simulink model "Test_Model_HR12_2016"  (R2016b)
settings: Solver=FixedStepAuto  StartTime=0.0  StopTime=length(ipoint)  FixedStep=dt  RelTol=1e-3
values from neighbouring files (symbols this model uses):
  Cbx_cyl_fill_efy_intk_mfld_prs_atm_prs_cor_cho = true    [Calib_mdl_RSA.m]
  Cbx_cyl_fill_efy_opt_cho = false    [Calib_mdl_RSA.m]
  Cbx_cyl_fill_igr_opt_cho = false    [Calib_mdl_RSA.m]
  Cbx_ex_vvt_conf = true    [Calib_mdl_RSA.m]
  Cnx_cyl_fill_ex_mfld_prs_cor_cho = 0    [Cal_basic.m]
  Cnx_cyl_nr_conf = 3    [Cal_basic.m]
  Cxx_cyl_fill_efy_drv_max = 20    [Calib_mdl_RSA.m]
  Cxx_cyl_fill_efy_dyn_max = 0.15    [Calib_mdl_RSA.m]
  Cxx_cyl_fill_efy_dyn_min = 0    [Calib_mdl_RSA.m]
  Cxx_cyl_fill_efy_dz = 0.45    [Calib_mdl_RSA.m]
  Cxx_cyl_fill_efy_ovlp_angl = 66    [Calib_mdl_RSA.m]
  Cxx_cyl_fill_efy_vvt_ofs = 0    [Calib_mdl_RSA.m]
  Cxx_cyl_fill_trap_area_h_thd = 0.2    [Cal_basic.m]
  Cxx_cyl_fill_trap_area_l_thd = 0.1    [Cal_basic.m]
  Cxx_cyl_fill_trap_efy_dz_l_thd = 1    [Cal_basic.m]
  Cxx_cyl_fill_trap_efy_dz_neg_slop = -0.5    [Cal_basic.m]
  Cxx_cyl_fill_trap_efy_dz_pos_slop = 0.5    [Cal_basic.m]
  Cxx_cyl_fill_trap_vvt_ovlp_angl = 120    [Calib_mdl_RSA.m]
  Cxx_cyl_vol = 3.9961e-04*3    (= 0.00119883)    [Cal_basic.m]    (also in Calib_mdl_RSA.m = 0.00119900004938)
  Cxx_min_cyl_fill_mdl_ex_mfld_prs_rat_cor = 0    [Cal_basic.m]
  Nnx_eng_run_stt = 2    [Calib_mdl_RSA.m]
  Nxx_atm_kpa = 101.3    [Cal_basic.m]
  Nxx_k_degc = 273.15    [Cal_basic.m]
  Nxx_kilo_bas = 1000    [Cal_basic.m]
  Nxx_wht_pgc_j_kg = 287    [Cal_basic.m]
undefined symbols (not defined in the file or in its folder): Cxx_egr_spc_heat, Cxx_thr_spc_heat, docblock, MapFilling_Aspirated
libraries: AEMS_Standard_Library x78, simulink x2
(part 3 of 5)

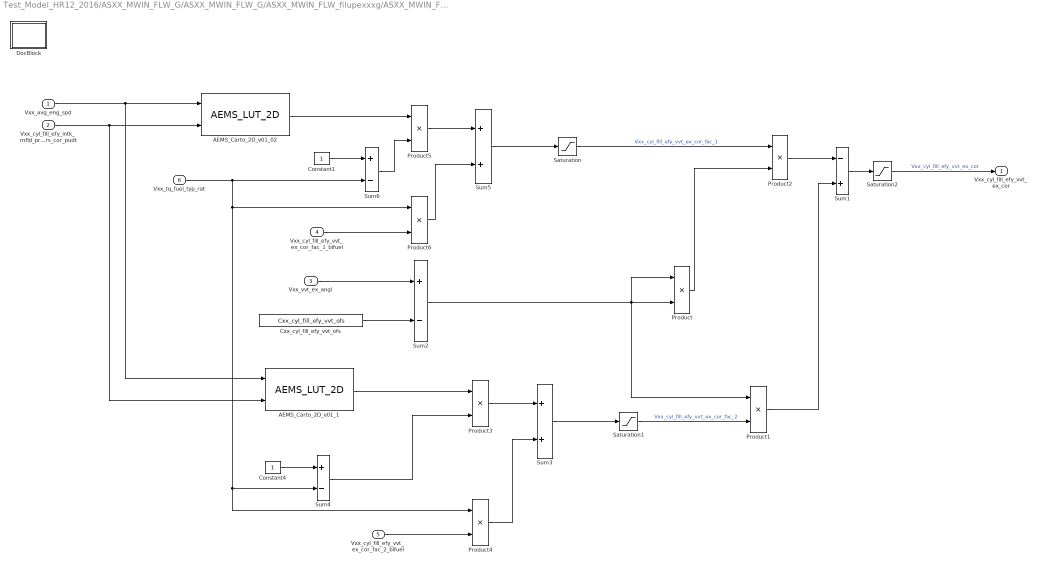
== system Test_Model_HR12_2016/ASXX_MWIN_FLW_G/ASXX_MWIN_FLW_G/ASXX_MWIN_FLW_filupexxxg/ASXX_MWIN_FLW_filupexxxg_10ms/Filupexxxg/B1_ex_parabolic_correction ==
  Vxx_avg_eng_spd : Inport  Interpolate=off
  Vxx_cyl_fill_efy_intk_mfld_prs_atm_prs_cor_pudt : Inport  Port=2  Interpolate=off
  Vxx_vvt_ex_angl : Inport  Port=3  Interpolate=off
  Vxx_cyl_fill_efy_vvt_ex_cor_fac_1_bifuel : Inport  Port=4  Interpolate=off
  Vxx_cyl_fill_efy_vvt_ex_cor_fac_2_bifuel : Inport  Port=5  Interpolate=off
  Vxx_tq_fuel_typ_rat : Inport  Port=6  Interpolate=off
  AEMS_Carto_2D_v01_02 : AEMS_Standard_Library/LOOKUP_TABLES/AEMS_LUT_2D  Tag=[LIB]  map_x=Cxb_cyl_fill_eng_spd  map_y=Cxb_cyl_fill_intk_mfld_prs  carto=Cxm_cyl_fill_efy_vvt_ex_cor_fac_1
      settings: AttributesFormatString=%<MaskType>\nBkPX=%<map_x>\nBkPY=%<map_y>\nMAP=%<carto>
  AEMS_Carto_2D_v01_1 : AEMS_Standard_Library/LOOKUP_TABLES/AEMS_LUT_2D  Tag=[LIB]  map_x=Cxb_cyl_fill_eng_spd  map_y=Cxb_cyl_fill_intk_mfld_prs  carto=Cxm_cyl_fill_efy_vvt_ex_cor_fac_2
      settings: AttributesFormatString=%<MaskType>\nBkPX=%<map_x>\nBkPY=%<map_y>\nMAP=%<carto>
  Constant1 : Constant
  Constant4 : Constant
  Cxx_cyl_fill_efy_vvt_ofs : Constant  Value=Cxx_cyl_fill_efy_vvt_ofs
  DocBlock : Subsystem  mask(DocBlock){ECoderFlag=, DocumentType=Text}
      mask prompts: ECoderFlag "Simulink:blocks:docblockEmbeddedCoderFlagLabel"; DocumentType "Simulink:blocks:docblockDocTypeLabel"
      mask help: Use this block to save long descriptive text with the model. Double-clicking the block will open an editor.
      mask TypeOptions DocumentType: Text | RTF | HTML
      mask Display:
      | plot([.8 0 0 1 1 .8 .8 1],[1 1 0 0 .8 1 .8 .8]);
      | text(.5,.6,'DOC','horizontalalignment','center');
      | text(.95,.05,get_param(gcb,'DocumentType'),'verticalalignment','bottom','horizontalalignment','right');
  Product{,1..6} (7 alike) : Product  OutDataTypeStr=Inherit: Inherit via back propagation  RndMeth=Zero
  Saturation : Saturate  UpperLimit=0.002000000094995  LowerLimit=-0.002000000094995  RndMeth=Zero
      settings: AttributesFormatString=<limits=%<UpperLimit>/%<LowerLimit>>
  Saturation1 : Saturate  UpperLimit=0.039062500000000  LowerLimit=-0.039062500000000  RndMeth=Zero
      settings: AttributesFormatString=<limits=%<UpperLimit>/%<LowerLimit>>
  Saturation2 : Saturate  UpperLimit=1  LowerLimit=-1  RndMeth=Zero
      settings: AttributesFormatString=<limits=%<UpperLimit>/%<LowerLimit>>
  Sum1 : Sum  Inputs=-+  OutDataTypeStr=Inherit: Inherit via back propagation  RndMeth=Zero  InputSameDT=on
  Sum2 : Sum  Inputs=+-  OutDataTypeStr=Inherit: Inherit via back propagation  RndMeth=Zero  InputSameDT=on
  Sum3 : Sum  OutDataTypeStr=Inherit: Inherit via back propagation  RndMeth=Zero  InputSameDT=on
  Sum4 : Sum  Inputs=+-  OutDataTypeStr=Inherit: Inherit via back propagation  RndMeth=Zero  InputSameDT=on
  Sum5 : Sum  OutDataTypeStr=Inherit: Inherit via back propagation  RndMeth=Zero  InputSameDT=on
  Sum6 : Sum  Inputs=+-  OutDataTypeStr=Inherit: Inherit via back propagation  RndMeth=Zero  InputSameDT=on
  Vxx_cyl_fill_efy_vvt_ex_cor : Outport
  wires:
  Vxx_vvt_ex_angl/1 -> Sum2/1
  Vxx_cyl_fill_efy_vvt_ex_cor_fac_1_bifuel/1 -> Product6/2
  Vxx_cyl_fill_efy_vvt_ex_cor_fac_2_bifuel/1 -> Product4/2
  Vxx_avg_eng_spd/1 -> AEMS_Carto_2D_v01_02/1, AEMS_Carto_2D_v01_1/1
  Vxx_cyl_fill_efy_intk_mfld_prs_atm_prs_cor_pudt/1 -> AEMS_Carto_2D_v01_02/2, AEMS_Carto_2D_v01_1/2
  Vxx_tq_fuel_typ_rat/1 -> Product4/1, Sum4/2, Product6/1, Sum6/2
  AEMS_Carto_2D_v01_02/1 -> Product5/1
  AEMS_Carto_2D_v01_1/1 -> Product3/1
  Constant1/1 -> Sum6/1
  Constant4/1 -> Sum4/1
  Product/1 -> Product2/2
  Product1/1 -> Sum1/2
  Product2/1 -> Sum1/1
  Product3/1 -> Sum3/1
  Product4/1 -> Sum3/2
  Product5/1 -> Sum5/1
  Product6/1 -> Sum5/2
  Sum1/1 -> Saturation2/1
  Sum2/1 -> Product/2, Product/1, Product1/1
  Sum3/1 -> Saturation1/1
  Sum4/1 -> Product3/2
  Sum5/1 -> Saturation/1
  Sum6/1 -> Product5/2
  Cxx_cyl_fill_efy_vvt_ofs/1 -> Sum2/2
  Saturation/1 -> Product2/1  "Vxx_cyl_fill_efy_vvt_ex_cor_fac_1"
  Saturation1/1 -> Product1/2  "Vxx_cyl_fill_efy_vvt_ex_cor_fac_2"
  Saturation2/1 -> Vxx_cyl_fill_efy_vvt_ex_cor/1  "Vxx_cyl_fill_efy_vvt_ex_cor"

== system Test_Model_HR12_2016/ASXX_MWIN_FLW_G/ASXX_MWIN_FLW_G/ASXX_MWIN_FLW_filupexxxg/ASXX_MWIN_FLW_filupexxxg_10ms/Filupexxxg/B2_overlap_correction ==
  Vxx_avg_eng_spd : Inport  Interpolate=off
  Vxx_cyl_fill_efy_intk_mfld_prs_atm_prs_cor_pudt : Inport  Port=2  Interpolate=off
  Vxx_vvt_intk_angl : Inport  Port=3  Interpolate=off
  Vxx_vvt_ex_angl : Inport  Port=4  Interpolate=off
  AEMS_Carto_2D_v01_02 : AEMS_Standard_Library/LOOKUP_TABLES/AEMS_LUT_2D  Tag=[LIB]  map_x=Cxb_cyl_fill_eng_spd  map_y=Cxb_cyl_fill_intk_mfld_prs  carto=Cxm_cyl_fill_efy_vvt_ovlp_cor_fac_1
      settings: AttributesFormatString=%<MaskType>\nBkPX=%<map_x>\nBkPY=%<map_y>\nMAP=%<carto>
  AEMS_Carto_2D_v01_1 : AEMS_Standard_Library/LOOKUP_TABLES/AEMS_LUT_2D  Tag=[LIB]  map_x=Cxb_cyl_fill_eng_spd  map_y=Cxb_cyl_fill_intk_mfld_prs  carto=Cxm_cyl_fill_efy_vvt_ovlp_cor_fac_2
      settings: AttributesFormatString=%<MaskType>\nBkPX=%<map_x>\nBkPY=%<map_y>\nMAP=%<carto>
  AEMS_Carto_2D_v01_2 : AEMS_Standard_Library/LOOKUP_TABLES/AEMS_LUT_2D  Tag=[LIB]  map_x=Cxb_cyl_fill_eng_spd  map_y=Cxb_cyl_fill_intk_mfld_prs  carto=Cxm_cyl_fill_efy_vvt_ovlp_cor_fac_3
      settings: AttributesFormatString=%<MaskType>\nBkPX=%<map_x>\nBkPY=%<map_y>\nMAP=%<carto>
  Constant4 : Constant  Value=0  OutDataTypeStr=single
  Cxx_cyl_fill_efy_ovlp_angl : Constant  Value=Cxx_cyl_fill_efy_ovlp_angl
  DocBlock : Subsystem  mask(DocBlock){ECoderFlag=, DocumentType=RTF}
      mask prompts: ECoderFlag "Simulink:blocks:docblockEmbeddedCoderFlagLabel"; DocumentType "Simulink:blocks:docblockDocTypeLabel"
      mask help: Use this block to save long descriptive text with the model. Double-clicking the block will open an editor.
      mask TypeOptions DocumentType: Text | RTF | HTML
      mask Display:
      | plot([.8 0 0 1 1 .8 .8 1],[1 1 0 0 .8 1 .8 .8]);
      | text(.5,.6,'DOC','horizontalalignment','center');
      | text(.95,.05,get_param(gcb,'DocumentType'),'verticalalignment','bottom','horizontalalignment','right');
  MinMax : MinMax  Function=max  Inputs=2  OutDataTypeStr=Inherit: Inherit via back propagation  RndMeth=Zero  InputSameDT=on
  Product : Product  OutDataTypeStr=Inherit: Inherit via back propagation  RndMeth=Zero
  Product1 : Product  Inputs=**  OutDataTypeStr=Inherit: Inherit via back propagation  RndMeth=Zero
  Product2 : Product  OutDataTypeStr=Inherit: Inherit via back propagation  RndMeth=Zero
  Product4 : Product  Inputs=**  OutDataTypeStr=Inherit: Inherit via back propagation  RndMeth=Zero
  Product5 : Product  Inputs=**  OutDataTypeStr=Inherit: Inherit via back propagation  RndMeth=Zero
  Saturation : Saturate  UpperLimit=1  LowerLimit=-1  RndMeth=Zero
      settings: AttributesFormatString=<limits=%<UpperLimit>/%<LowerLimit>>
  Sum1 : Sum  OutDataTypeStr=Inherit: Inherit via back propagation  RndMeth=Zero  InputSameDT=on
  Sum2 : Sum  Inputs=+-  OutDataTypeStr=Inherit: Inherit via back propagation  RndMeth=Zero  InputSameDT=on
  Sum3 : Sum  OutDataTypeStr=Inherit: Inherit via back propagation  RndMeth=Zero  InputSameDT=on
  Sum4 : Sum  OutDataTypeStr=Inherit: Inherit via back propagation  RndMeth=Zero  InputSameDT=on
  Vxx_cyl_fill_efy_vvt_ovlp_cor : Outport
  wires:
  Vxx_vvt_intk_angl/1 -> Sum3/1
  Vxx_vvt_ex_angl/1 -> Sum3/2
  Vxx_avg_eng_spd/1 -> AEMS_Carto_2D_v01_2/1, AEMS_Carto_2D_v01_1/1, AEMS_Carto_2D_v01_02/1
  Vxx_cyl_fill_efy_intk_mfld_prs_atm_prs_cor_pudt/1 -> AEMS_Carto_2D_v01_02/2, AEMS_Carto_2D_v01_2/2, AEMS_Carto_2D_v01_1/2
  AEMS_Carto_2D_v01_02/1 -> Product/1  "Vxx_cyl_fill_efy_vvt_ovlp_cor_fac_1"
  AEMS_Carto_2D_v01_1/1 -> Product1/2  "Vxx_cyl_fill_efy_vvt_ovlp_cor_fac_2"
  AEMS_Carto_2D_v01_2/1 -> Product5/2  "Vxx_cyl_fill_efy_vvt_ovlp_cor_fac_3"
  Constant4/1 -> MinMax/2
  Cxx_cyl_fill_efy_ovlp_angl/1 -> Sum2/2
  MinMax/1 -> Product2/1, Product5/1, Product4/2, Product4/1
  Product/1 -> Sum1/1
  Product1/1 -> Sum1/2
  Product2/1 -> Product/2
  Product4/1 -> Product1/1, Product2/2
  Product5/1 -> Sum4/2
  Saturation/1 -> Vxx_cyl_fill_efy_vvt_ovlp_cor/1  "Vxx_cyl_fill_efy_vvt_ovlp_cor"
  Sum1/1 -> Sum4/1
  Sum2/1 -> MinMax/1
  Sum3/1 -> Sum2/1
  Sum4/1 -> Saturation/1

== system Test_Model_HR12_2016/ASXX_MWIN_FLW_G/ASXX_MWIN_FLW_G/ASXX_MWIN_FLW_filupxxxxg/ASXX_MWIN_FLW_filupxxxxg_10ms/A_Parabolic_model/A1_altimetric_correction ==
  Vxx_intk_mfld_prs : Inport  Interpolate=off
  Vxx_atm_prs : Inport  Port=2  Interpolate=off
  Cbx_vvtc_alti_cor_map_cfm : Constant  Value=Cbx_cyl_fill_efy_intk_mfld_prs_atm_prs_cor_cho
  DocBlock : Subsystem  mask(DocBlock){ECoderFlag=, DocumentType=Text}
      mask prompts: ECoderFlag "Simulink:blocks:docblockEmbeddedCoderFlagLabel"; DocumentType "Simulink:blocks:docblockDocTypeLabel"
      mask help: Use this block to save long descriptive text with the model. Double-clicking the block will open an editor.
      mask TypeOptions DocumentType: Text | RTF | HTML
      mask Display:
      | plot([.8 0 0 1 1 .8 .8 1],[1 1 0 0 .8 1 .8 .8]);
      | text(.5,.6,'DOC','horizontalalignment','center');
      | text(.95,.05,get_param(gcb,'DocumentType'),'verticalalignment','bottom','horizontalalignment','right');
  Nxx_atm_hpa : Constant  Value=Nxx_atm_kpa
  Saturation8 : Saturate  UpperLimit=2000  LowerLimit=0  RndMeth=Zero
      settings: AttributesFormatString=<limits=%<UpperLimit>/%<LowerLimit>>
  Sum6 : Sum  Inputs=+-  OutDataTypeStr=Inherit: Inherit via back propagation  RndMeth=Zero  InputSameDT=on
  Sum7 : Sum  OutDataTypeStr=Inherit: Inherit via back propagation  RndMeth=Zero  InputSameDT=on
  Switch1 : Switch  Criteria=u2 ~= 0  RndMeth=Zero  SaturateOnIntegerOverflow=on  InputSameDT=on
      settings: AttributesFormatString=Criteria=%<Criteria>
  Vxx_cyl_fill_efy_intk_mfld_prs_atm_prs_cor : Outport
  wires:
  Switch1/1 -> Saturation8/1
  Vxx_atm_prs/1 -> Sum6/2
  Nxx_atm_hpa/1 -> Sum6/1
  Sum6/1 -> Sum7/2
  Sum7/1 -> Switch1/3
  Cbx_vvtc_alti_cor_map_cfm/1 -> Switch1/2
  Vxx_intk_mfld_prs/1 -> Switch1/1, Sum7/1
  Saturation8/1 -> Vxx_cyl_fill_efy_intk_mfld_prs_atm_prs_cor/1  "Vxx_cyl_fill_efy_intk_mfld_prs_atm_prs_cor"

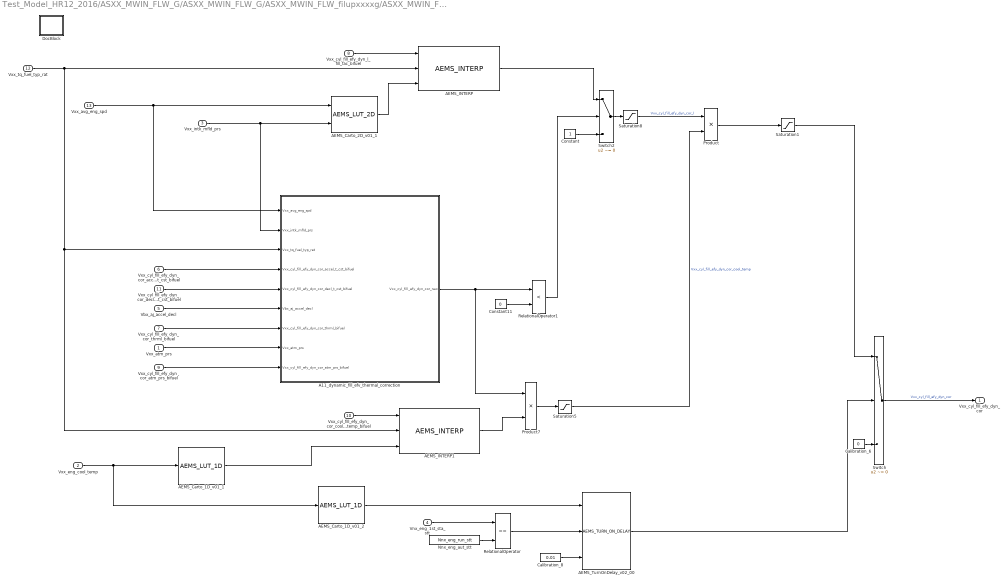
== system Test_Model_HR12_2016/ASXX_MWIN_FLW_G/ASXX_MWIN_FLW_G/ASXX_MWIN_FLW_filupxxxxg/ASXX_MWIN_FLW_filupxxxxg_10ms/A_Parabolic_model/A2_dynamic_fill_efv ==
  Vxx_atm_prs : Inport  Interpolate=off
  Vxx_eng_cool_temp : Inport  Port=2  Interpolate=off
  Vxx_intk_mfld_prs : Inport  Port=3  Interpolate=off
  Vnx_eng_1st_sta_stt : Inport  Port=4  Interpolate=off
  Vbx_aj_accel_decl : Inport  Port=5  Interpolate=off
  Vxx_cyl_fill_efy_dyn_cor_accel_t_cst_bifuel : Inport  Port=6  Interpolate=off
  Vxx_cyl_fill_efy_dyn_cor_thrml_bifuel : Inport  Port=7  Interpolate=off
  Vxx_cyl_fill_efy_dyn_l_fill_fac_bifuel : Inport  Port=8  Interpolate=off
  Vxx_cyl_fill_efy_dyn_cor_atm_prs_bifuel : Inport  Port=9  Interpolate=off
  Vxx_cyl_fill_efy_dyn_cor_cool_temp_bifuel : Inport  Port=10  Interpolate=off
  Vxx_cyl_fill_efy_dyn_cor_decl_t_cst_bifuel : Inport  Port=11  Interpolate=off
  Vxx_tq_fuel_typ_rat : Inport  Port=12  Interpolate=off
  Vxx_avg_eng_spd : Inport  Port=13  Interpolate=off
  A11_dynamic_fill_efv_thermal_correction : Subsystem
  AEMS_Carto_1D_v01_1 : AEMS_Standard_Library/LOOKUP_TABLES/AEMS_LUT_1D  Tag=[LIB]  map_x=Cxb_eng_cool_temp_2  map_z=Cxp_cyl_fill_efy_dyn_cor_cool_temp
      settings: AttributesFormatString=%<MaskType>\nBkPX=%<map_x>\nLUT=%<map_z>
  AEMS_Carto_1D_v01_2 : AEMS_Standard_Library/LOOKUP_TABLES/AEMS_LUT_1D  Tag=[LIB]  map_x=Cxb_eng_cool_temp_2  map_z=Cxp_cyl_fill_efy_dyn_off_dly
      settings: AttributesFormatString=%<MaskType>\nBkPX=%<map_x>\nLUT=%<map_z>
  AEMS_Carto_2D_v01_1 : AEMS_Standard_Library/LOOKUP_TABLES/AEMS_LUT_2D  Tag=[LIB]  map_x=Cxb_cyl_fill_eng_spd  map_y=Cxb_cyl_fill_intk_mfld_prs  carto=Cxm_cyl_fill_efy_dyn_l_fill_fac
      settings: AttributesFormatString=%<MaskType>\nBkPX=%<map_x>\nBkPY=%<map_y>\nMAP=%<carto>
  AEMS_INTERP : AEMS_Standard_Library/LOOKUP_TABLES/AEMS_INTERP  Tag=[LIB]  Description=This library calculates interpolation for 2 inputs.
      settings: AttributesFormatString=%<MaskType>
  AEMS_INTERP1 : AEMS_Standard_Library/LOOKUP_TABLES/AEMS_INTERP  Tag=[LIB]  Description=This library calculates interpolation for 2 inputs.
      settings: AttributesFormatString=%<MaskType>
  AEMS_TurnOnDelay_v02_00 : AEMS_Standard_Library/TIMER/AEMS_TURN_ON_DELAY  Tag=[LIB]  timeoutinit=0  initinit=0
      settings: AttributesFormatString=%<MaskType>\nOutput initialization=%<timeoutinit>\nInput initialization=%<initinit>
  Calibration_6 : Constant  Value=0
  Calibration_8 : Constant  Value=0.01
  Constant : Constant
  Constant11 : Constant  Value=0
  DocBlock : Subsystem  mask(DocBlock){ECoderFlag=, DocumentType=Text}
      mask prompts: ECoderFlag "Simulink:blocks:docblockEmbeddedCoderFlagLabel"; DocumentType "Simulink:blocks:docblockDocTypeLabel"
      mask help: Use this block to save long descriptive text with the model. Double-clicking the block will open an editor.
      mask TypeOptions DocumentType: Text | RTF | HTML
      mask Display:
      | plot([.8 0 0 1 1 .8 .8 1],[1 1 0 0 .8 1 .8 .8]);
      | text(.5,.6,'DOC','horizontalalignment','center');
      | text(.95,.05,get_param(gcb,'DocumentType'),'verticalalignment','bottom','horizontalalignment','right');
  Nnx_eng_aut_stt : Constant  Value=Nnx_eng_run_stt
  Product : Product  OutDataTypeStr=Inherit: Inherit via back propagation  RndMeth=Zero
  Product7 : Product  OutDataTypeStr=Inherit: Inherit via back propagation  RndMeth=Zero
  RelationalOperator : RelationalOperator  Operator===  OutDataTypeStr=boolean  RndMeth=Nearest  InputSameDT=on
  RelationalOperator1 : RelationalOperator  Operator=<  OutDataTypeStr=boolean  RndMeth=Nearest  InputSameDT=on
  Saturation1 : Saturate  UpperLimit=Cxx_cyl_fill_efy_dyn_max  LowerLimit=Cxx_cyl_fill_efy_dyn_min  RndMeth=Zero
      settings: AttributesFormatString=<limits=%<UpperLimit>/%<LowerLimit>>
  Saturation5 : Saturate  UpperLimit=1  LowerLimit=-1  RndMeth=Zero
      settings: AttributesFormatString=<limits=%<UpperLimit>/%<LowerLimit>>
  Saturation8 : Saturate  UpperLimit=2  LowerLimit=0  RndMeth=Zero
      settings: AttributesFormatString=<limits=%<UpperLimit>/%<LowerLimit>>
  Switch : Switch  Criteria=u2 ~= 0  RndMeth=Zero  SaturateOnIntegerOverflow=on  InputSameDT=on
      settings: AttributesFormatString=Criteria=%<Criteria>
  Switch2 : Switch  Criteria=u2 ~= 0  RndMeth=Zero  SaturateOnIntegerOverflow=on  InputSameDT=on
      settings: AttributesFormatString=Criteria=%<Criteria>
  Vxx_cyl_fill_efy_dyn_cor : Outport
  wires:
  Switch/1 -> Vxx_cyl_fill_efy_dyn_cor/1  "Vxx_cyl_fill_efy_dyn_cor"
  Vxx_cyl_fill_efy_dyn_cor_cool_temp_bifuel/1 -> AEMS_INTERP1/1
  Vxx_cyl_fill_efy_dyn_l_fill_fac_bifuel/1 -> AEMS_INTERP/1
  Vnx_eng_1st_sta_stt/1 -> RelationalOperator/1
  Vxx_eng_cool_temp/1 -> AEMS_Carto_1D_v01_2/1, AEMS_Carto_1D_v01_1/1
  Nnx_eng_aut_stt/1 -> RelationalOperator/2
  Constant11/1 -> RelationalOperator1/2
  Constant/1 -> Switch2/3
  Calibration_8/1 -> AEMS_TurnOnDelay_v02_00/3
  Calibration_6/1 -> Switch/3
  AEMS_Carto_2D_v01_1/1 -> AEMS_INTERP/3
  Saturation1/1 -> Switch/1
  Product7/1 -> Saturation5/1
  Switch2/1 -> Saturation8/1
  AEMS_TurnOnDelay_v02_00/1 -> Switch/2
  RelationalOperator/1 -> AEMS_TurnOnDelay_v02_00/2
  Product/1 -> Saturation1/1
  RelationalOperator1/1 -> Switch2/2
  AEMS_Carto_1D_v01_2/1 -> AEMS_TurnOnDelay_v02_00/1
  Vxx_tq_fuel_typ_rat/1 -> AEMS_INTERP1/2, A11_dynamic_fill_efv_thermal_correction/3(Vxx_tq_fuel_typ_rat), AEMS_INTERP/2
  Vxx_avg_eng_spd/1 -> A11_dynamic_fill_efv_thermal_correction/1(Vxx_avg_eng_spd), AEMS_Carto_2D_v01_1/1
  Vxx_intk_mfld_prs/1 -> A11_dynamic_fill_efv_thermal_correction/2(Vxx_intk_mfld_prs), AEMS_Carto_2D_v01_1/2
  Saturation8/1 -> Product/1  "Vxx_cyl_fill_efy_dyn_cor_l"
  Saturation5/1 -> Product/2  "Vxx_cyl_fill_efy_dyn_cor_cool_temp"
  A11_dynamic_fill_efv_thermal_correction/1(Vxx_cyl_fill_efy_dyn_cor_raw) -> Product7/1, RelationalOperator1/1
  Vxx_cyl_fill_efy_dyn_cor_accel_t_cst_bifuel/1 -> A11_dynamic_fill_efv_thermal_correction/4(Vxx_cyl_fill_efy_dyn_cor_accel_t_cst_bifuel)
  Vxx_cyl_fill_efy_dyn_cor_decl_t_cst_bifuel/1 -> A11_dynamic_fill_efv_thermal_correction/5(Vxx_cyl_fill_efy_dyn_cor_decl_t_cst_bifuel)
  Vbx_aj_accel_decl/1 -> A11_dynamic_fill_efv_thermal_correction/6(Vbx_aj_accel_decl)
  Vxx_cyl_fill_efy_dyn_cor_thrml_bifuel/1 -> A11_dynamic_fill_efv_thermal_correction/7(Vxx_cyl_fill_efy_dyn_cor_thrml_bifuel)
  Vxx_atm_prs/1 -> A11_dynamic_fill_efv_thermal_correction/8(Vxx_atm_prs)
  Vxx_cyl_fill_efy_dyn_cor_atm_prs_bifuel/1 -> A11_dynamic_fill_efv_thermal_correction/9(Vxx_cyl_fill_efy_dyn_cor_atm_prs_bifuel)
  AEMS_Carto_1D_v01_1/1 -> AEMS_INTERP1/3
  AEMS_INTERP/1 -> Switch2/1
  AEMS_INTERP1/1 -> Product7/2

== system Test_Model_HR12_2016/ASXX_MWIN_FLW_G/ASXX_MWIN_FLW_G/ASXX_MWIN_FLW_filupxxxxg/ASXX_MWIN_FLW_filupxxxxg_10ms/A_Parabolic_model/A3_fil_efv_cylndr_deactivate ==
  Vxx_avg_eng_spd : Inport  Interpolate=off
  Vxx_intk_mfld_prs : Inport  Port=2  Interpolate=off
  Vxx_cyl_fill_efy_bas_bifuel : Inport  Port=3  Interpolate=off
  Vxx_tq_fuel_typ_rat : Inport  Port=4  Interpolate=off
  AEMS_Carto_2D_v01_02 : AEMS_Standard_Library/LOOKUP_TABLES/AEMS_LUT_2D  Tag=[LIB]  map_x=Cxb_cyl_fill_eng_spd  map_y=Cxb_cyl_fill_intk_mfld_prs  carto=Cxm_cyl_fill_efy_bas
      settings: AttributesFormatString=%<MaskType>\nBkPX=%<map_x>\nBkPY=%<map_y>\nMAP=%<carto>
  AEMS_INTERP : AEMS_Standard_Library/LOOKUP_TABLES/AEMS_INTERP  Tag=[LIB]  Description=This library calculates interpolation for 2 inputs.
      settings: AttributesFormatString=%<MaskType>
  AEMS_LUT_2D : AEMS_Standard_Library/LOOKUP_TABLES/AEMS_LUT_2D  Tag=[LIB]  map_x=Cxb_cyl_fill_eng_spd  map_y=Cxb_cyl_fill_intk_mfld_prs  carto=Cxm_cyl_fill_efy_bas_vvl_intk_l_lift
      settings: AttributesFormatString=%<MaskType>\nBkPX=%<map_x>\nBkPY=%<map_y>\nMAP=%<carto>
  Data Type Conversion2 : DataTypeConversion
  DocBlock : Subsystem  mask(DocBlock){ECoderFlag=, DocumentType=Text}
      mask prompts: ECoderFlag "Simulink:blocks:docblockEmbeddedCoderFlagLabel"; DocumentType "Simulink:blocks:docblockDocTypeLabel"
      mask help: Use this block to save long descriptive text with the model. Double-clicking the block will open an editor.
      mask TypeOptions DocumentType: Text | RTF | HTML
      mask Display:
      | plot([.8 0 0 1 1 .8 .8 1],[1 1 0 0 .8 1 .8 .8]);
      | text(.5,.6,'DOC','horizontalalignment','center');
      | text(.95,.05,get_param(gcb,'DocumentType'),'verticalalignment','bottom','horizontalalignment','right');
  Mux : Mux  Inputs=2
  Saturation8 : Saturate  UpperLimit=2  LowerLimit=0  RndMeth=Zero
      settings: AttributesFormatString=<limits=%<UpperLimit>/%<LowerLimit>>
  Vxt_cyl_fill_efy_bas : Outport
  wires:
  Vxx_intk_mfld_prs/1 -> AEMS_LUT_2D/2, AEMS_Carto_2D_v01_02/2
  Vxx_avg_eng_spd/1 -> AEMS_LUT_2D/1, AEMS_Carto_2D_v01_02/1
  Mux/1 -> Data Type Conversion2/1
  Vxx_cyl_fill_efy_bas_bifuel/1 -> AEMS_INTERP/1
  Vxx_tq_fuel_typ_rat/1 -> AEMS_INTERP/2
  AEMS_INTERP/1 -> Saturation8/1
  AEMS_LUT_2D/1 -> Mux/2
  AEMS_Carto_2D_v01_02/1 -> Mux/1
  Data Type Conversion2/1 -> AEMS_INTERP/3  "Vxt_cyl_fill_efy_temp"
  Saturation8/1 -> Vxt_cyl_fill_efy_bas/1  "Vxt_cyl_fill_efy_bas"

== system Test_Model_HR12_2016/ASXX_MWIN_FLW_G/ASXX_MWIN_FLW_G/ASXX_MWIN_FLW_filupxxxxg/ASXX_MWIN_FLW_filupxxxxg_10ms/A_Parabolic_model/A4_adm_parabolic_correction ==
  Vxx_cyl_fill_efy_intk_mfld_prs_atm_prs_cor : Inport  Interpolate=off
  Vxx_avg_eng_spd : Inport  Port=2  Interpolate=off
  Vxx_vvt_intk_angl : Inport  Port=3  Interpolate=off
  Vxx_tq_fuel_typ_rat : Inport  Port=4  Interpolate=off
  Vxx_cyl_fill_efy_vvt_intk_cor_fac_1_bifuel : Inport  Port=5  Interpolate=off
  Vxx_cyl_fill_efy_vvt_intk_cor_fac_2_bifuel : Inport  Port=6  Interpolate=off
  AEMS_Carto_2D_v01_1 : AEMS_Standard_Library/LOOKUP_TABLES/AEMS_LUT_2D  Tag=[LIB]  map_x=Cxb_cyl_fill_eng_spd  map_y=Cxb_cyl_fill_intk_mfld_prs  carto=Cxm_cyl_fill_efy_vvt_cor_fac_2
      settings: AttributesFormatString=%<MaskType>\nBkPX=%<map_x>\nBkPY=%<map_y>\nMAP=%<carto>
  AEMS_Carto_2D_v01_2 : AEMS_Standard_Library/LOOKUP_TABLES/AEMS_LUT_2D  Tag=[LIB]  map_x=Cxb_cyl_fill_eng_spd  map_y=Cxb_cyl_fill_intk_mfld_prs  carto=Cxm_cyl_fill_efy_vvt_cor_fac_1
      settings: AttributesFormatString=%<MaskType>\nBkPX=%<map_x>\nBkPY=%<map_y>\nMAP=%<carto>
  AEMS_Carto_2D_v01_3 : AEMS_Standard_Library/LOOKUP_TABLES/AEMS_LUT_2D  Tag=[LIB]  map_x=Cxb_cyl_fill_eng_spd  map_y=Cxb_cyl_fill_intk_mfld_prs  carto=Cxm_cyl_fill_efy_vvt_cor_fac_2_vvl_intk_l_lift
      settings: AttributesFormatString=%<MaskType>\nBkPX=%<map_x>\nBkPY=%<map_y>\nMAP=%<carto>
  AEMS_Carto_2D_v01_4 : AEMS_Standard_Library/LOOKUP_TABLES/AEMS_LUT_2D  Tag=[LIB]  map_x=Cxb_cyl_fill_eng_spd  map_y=Cxb_cyl_fill_intk_mfld_prs  carto=Cxm_cyl_fill_efy_vvt_cor_fac_1_vvl_intk_l_lift
      settings: AttributesFormatString=%<MaskType>\nBkPX=%<map_x>\nBkPY=%<map_y>\nMAP=%<carto>
  AEMS_INTERP : AEMS_Standard_Library/LOOKUP_TABLES/AEMS_INTERP  Tag=[LIB]  Description=This library calculates interpolation for 2 inputs.
      settings: AttributesFormatString=%<MaskType>
  AEMS_INTERP1 : AEMS_Standard_Library/LOOKUP_TABLES/AEMS_INTERP  Tag=[LIB]  Description=This library calculates interpolation for 2 inputs.
      settings: AttributesFormatString=%<MaskType>
  Cxx_cyl_fill_efy_vvt_ofs : Constant  Value=Cxx_cyl_fill_efy_vvt_ofs
  DocBlock : Subsystem  mask(DocBlock){ECoderFlag=, DocumentType=RTF}
      mask prompts: ECoderFlag "Simulink:blocks:docblockEmbeddedCoderFlagLabel"; DocumentType "Simulink:blocks:docblockDocTypeLabel"
      mask help: Use this block to save long descriptive text with the model. Double-clicking the block will open an editor.
      mask TypeOptions DocumentType: Text | RTF | HTML
      mask Display:
      | plot([.8 0 0 1 1 .8 .8 1],[1 1 0 0 .8 1 .8 .8]);
      | text(.5,.6,'DOC','horizontalalignment','center');
      | text(.95,.05,get_param(gcb,'DocumentType'),'verticalalignment','bottom','horizontalalignment','right');
  Mux : Mux  Inputs=2
  Mux1 : Mux  Inputs=2
  Product1 : Product  OutDataTypeStr=Inherit: Inherit via back propagation  RndMeth=Zero
  Product2 : Product  OutDataTypeStr=Inherit: Inherit via back propagation  RndMeth=Zero
  Product3 : Product  OutDataTypeStr=Inherit: Inherit via back propagation  RndMeth=Zero
  Saturation : Saturate  UpperLimit=1  LowerLimit=-1  RndMeth=Zero
      settings: AttributesFormatString=<limits=%<UpperLimit>/%<LowerLimit>>
  Saturation1 : Saturate  UpperLimit=0.0390625  LowerLimit=-0.0390625  RndMeth=Zero
      settings: AttributesFormatString=<limits=%<UpperLimit>/%<LowerLimit>>
  Saturation8 : Saturate  UpperLimit=0.0390625  LowerLimit=-0.0390625  RndMeth=Zero
      settings: AttributesFormatString=<limits=%<UpperLimit>/%<LowerLimit>>
  Sum1 : Sum  Inputs=-+  OutDataTypeStr=Inherit: Inherit via back propagation  RndMeth=Zero  InputSameDT=on
  Sum2 : Sum  Inputs=+-  OutDataTypeStr=Inherit: Inherit via back propagation  RndMeth=Zero  InputSameDT=on
  Vxt_cyl_fill_efy_vvt_intk_cor : Outport
  wires:
  Saturation/1 -> Vxt_cyl_fill_efy_vvt_intk_cor/1  "Vxt_cyl_fill_efy_vvt_intk_cor"
  Product1/1 -> Sum1/2
  Cxx_cyl_fill_efy_vvt_ofs/1 -> Sum2/2
  Sum2/1 -> Product2/2, Product3/2, Product1/1
  Sum1/1 -> Saturation/1
  Product3/1 -> Sum1/1
  Product2/1 -> Product3/1
  Vxx_vvt_intk_angl/1 -> Sum2/1
  Vxx_tq_fuel_typ_rat/1 -> AEMS_INTERP/2, AEMS_INTERP1/2
  Vxx_cyl_fill_efy_vvt_intk_cor_fac_1_bifuel/1 -> AEMS_INTERP/1
  Vxx_cyl_fill_efy_vvt_intk_cor_fac_2_bifuel/1 -> AEMS_INTERP1/1
  Vxx_avg_eng_spd/1 -> AEMS_Carto_2D_v01_4/1, AEMS_Carto_2D_v01_2/1, AEMS_Carto_2D_v01_1/1, AEMS_Carto_2D_v01_3/1
  Vxx_cyl_fill_efy_intk_mfld_prs_atm_prs_cor/1 -> AEMS_Carto_2D_v01_4/2, AEMS_Carto_2D_v01_2/2, AEMS_Carto_2D_v01_1/2, AEMS_Carto_2D_v01_3/2
  AEMS_Carto_2D_v01_2/1 -> Mux/1
  AEMS_Carto_2D_v01_4/1 -> Mux/2
  Mux/1 -> AEMS_INTERP/3
  AEMS_Carto_2D_v01_1/1 -> Mux1/1
  AEMS_Carto_2D_v01_3/1 -> Mux1/2
  Mux1/1 -> AEMS_INTERP1/3
  Saturation8/1 -> Product2/1  "Vxt_cyl_fill_efy_vvt_intk_cor_fac_1"
  Saturation1/1 -> Product1/2  "Vxt_cyl_fill_efy_vvt_intk_cor_fac_2"
  AEMS_INTERP/1 -> Saturation8/1
  AEMS_INTERP1/1 -> Saturation1/1

== system Test_Model_HR12_2016/ASXX_MWIN_FLW_G/ASXX_MWIN_FLW_G/ASXX_MWIN_FLW_filupxxxxg/ASXX_MWIN_FLW_filupxxxxg_10ms/A_Parabolic_model/A5_vlv_air_temp_correction ==
  Vxx_intk_vlv_temp : Inport  Interpolate=off
  Vxx_cyl_fill_efy_temp_cor_bifuel : Inport  Port=2  Interpolate=off
  Vxx_intk_mfld_prs : Inport  Port=3  Interpolate=off
  Vxx_tq_fuel_typ_rat : Inport  Port=4  Interpolate=off
  AEMS_Carto_2D_v01_02 : AEMS_Standard_Library/LOOKUP_TABLES/AEMS_LUT_2D  Tag=[LIB]  map_x=Cxb_intk_mfld_temp_2  map_y=Cxb_cyl_fill_intk_mfld_prs  carto=Cxm_cyl_fill_efy_intk_vlv_temp_cor
      settings: AttributesFormatString=%<MaskType>\nBkPX=%<map_x>\nBkPY=%<map_y>\nMAP=%<carto>
  AEMS_INTERP : AEMS_Standard_Library/LOOKUP_TABLES/AEMS_INTERP  Tag=[LIB]  Description=This library calculates interpolation for 2 inputs.
      settings: AttributesFormatString=%<MaskType>
  DocBlock : Subsystem  mask(DocBlock){ECoderFlag=, DocumentType=Text}
      mask prompts: ECoderFlag "Simulink:blocks:docblockEmbeddedCoderFlagLabel"; DocumentType "Simulink:blocks:docblockDocTypeLabel"
      mask help: Use this block to save long descriptive text with the model. Double-clicking the block will open an editor.
      mask TypeOptions DocumentType: Text | RTF | HTML
      mask Display:
      | plot([.8 0 0 1 1 .8 .8 1],[1 1 0 0 .8 1 .8 .8]);
      | text(.5,.6,'DOC','horizontalalignment','center');
      | text(.95,.05,get_param(gcb,'DocumentType'),'verticalalignment','bottom','horizontalalignment','right');
  Saturation8 : Saturate  UpperLimit=2  LowerLimit=0  RndMeth=Zero
      settings: AttributesFormatString=<limits=%<UpperLimit>/%<LowerLimit>>
  Vxx_cyl_fill_efy_temp_cor : Outport
  wires:
  Vxx_intk_vlv_temp/1 -> AEMS_Carto_2D_v01_02/1
  Vxx_intk_mfld_prs/1 -> AEMS_Carto_2D_v01_02/2
  AEMS_Carto_2D_v01_02/1 -> AEMS_INTERP/3
  AEMS_INTERP/1 -> Saturation8/1
  Vxx_tq_fuel_typ_rat/1 -> AEMS_INTERP/2
  Vxx_cyl_fill_efy_temp_cor_bifuel/1 -> AEMS_INTERP/1
  Saturation8/1 -> Vxx_cyl_fill_efy_temp_cor/1  "Vxx_cyl_fill_efy_temp_cor"

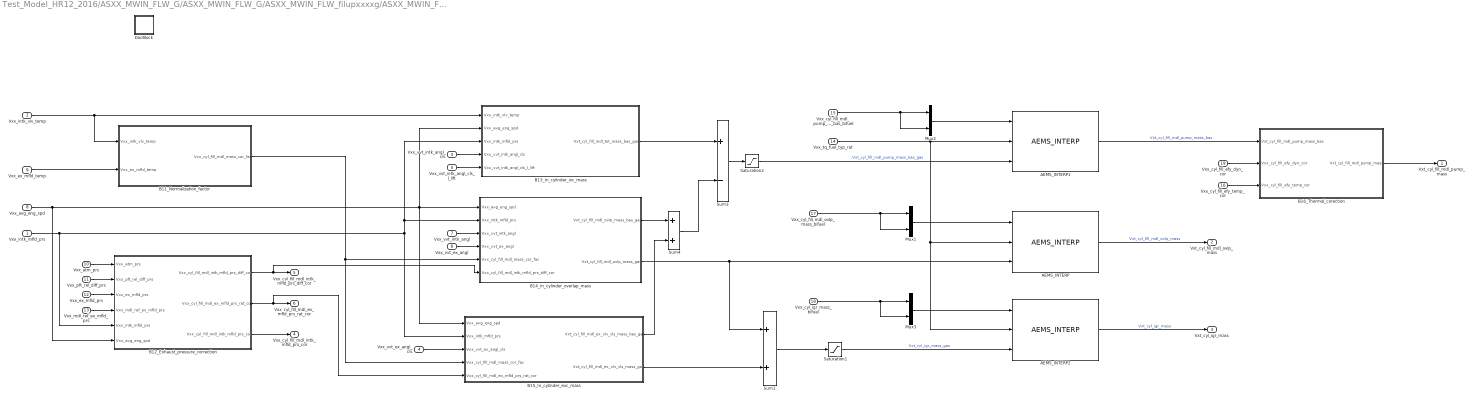
== system Test_Model_HR12_2016/ASXX_MWIN_FLW_G/ASXX_MWIN_FLW_G/ASXX_MWIN_FLW_filupxxxxg/ASXX_MWIN_FLW_filupxxxxg_10ms/B_Optional_air_filling_estimation/B1_Pumped_mass_caculation ==
  Vxx_intk_mfld_prs : Inport  Interpolate=off
  Vxx_intk_vlv_temp : Inport  Port=2  Interpolate=off
  Vxx_vvt_intk_angl_cls : Inport  Port=3  Interpolate=off
  Vxx_vvt_ex_angl_cls : Inport  Port=4  Interpolate=off
  Vxx_vvt_intk_angl_cls_l_lift : Inport  Port=5  Interpolate=off
  Vxx_vvt_ex_angl : Inport  Port=6  Interpolate=off
  Vxx_vvt_intk_angl : Inport  Port=7  Interpolate=off
  Vxx_avg_eng_spd : Inport  Port=8  Interpolate=off
  Vxx_ex_mfld_temp : Inport  Port=9  Interpolate=off
  Vxx_atm_prs : Inport  Port=10  Interpolate=off
  Vxx_pft_rel_diff_prs : Inport  Port=11  Interpolate=off
  Vxx_ex_mfld_prs : Inport  Port=12  Interpolate=off
  Vxx_mdl_ref_ex_mfld_prs : Inport  Port=13  Interpolate=off
  Vxx_tq_fuel_typ_rat : Inport  Port=14  Interpolate=off
  Vxx_cyl_fill_mdl_pump_mass_bas_bifuel : Inport  Port=15  Interpolate=off
  Vxx_cyl_fill_efy_temp_cor : Inport  Port=16  Interpolate=off
  Vxx_cyl_fill_mdl_ovlp_mass_bifuel : Inport  Port=17  Interpolate=off
  Vxx_cyl_igr_mass_bifuel : Inport  Port=18  Interpolate=off
  Vxx_cyl_fill_efy_dyn_cor : Inport  Port=19  Interpolate=off
  AEMS_INTERP : AEMS_Standard_Library/LOOKUP_TABLES/AEMS_INTERP  Tag=[LIB]  Description=This library calculates interpolation for 2 inputs.
      settings: AttributesFormatString=%<MaskType>
  AEMS_INTERP1 : AEMS_Standard_Library/LOOKUP_TABLES/AEMS_INTERP  Tag=[LIB]  Description=This library calculates interpolation for 2 inputs.
      settings: AttributesFormatString=%<MaskType>
  AEMS_INTERP2 : AEMS_Standard_Library/LOOKUP_TABLES/AEMS_INTERP  Tag=[LIB]  Description=This library calculates interpolation for 2 inputs.
      settings: AttributesFormatString=%<MaskType>
  B11_Normalization_factor : Subsystem
  B12_Exhaust_pressure_correction : Subsystem
  B13_In_cylinder_ivc_mass : Subsystem
  B14_In_cylinder_overlap_mass : Subsystem
  B15_In_cylinder_evc_mass : Subsystem
  B16_Thermal_corection : Subsystem
  DocBlock : Subsystem  InitFcn=docblock('save_document',gcb);  mask(DocBlock){ECoderFlag=, DocumentType=RTF}
      mask prompts: ECoderFlag "Simulink:masks:DocBlockEmbeddedCoderFlagLabel_MP"; DocumentType "Simulink:masks:DocBlockDocTypeLabel_MP"
      mask help: Simulink:masks:DocBlock_MD
      settings: DeleteFcn=docblock('close_document',gcb);  PreSaveFcn=docblock('save_document',gcb);  OpenFcn=docblock('edit_document',gcb);
      mask TypeOptions DocumentType: Simulink:masks:Text | Simulink:masks:RTF | Simulink:masks:HTML
      mask Display:
      | plot([.8 0 0 1 1 .8 .8 1],[1 1 0 0 .8 1 .8 .8]);
      | text(.5,.6,'DOC','horizontalalignment','center');
      | text(.95,.05,get_param(gcb,'DocumentType'),'verticalalignment','bottom','horizontalalignment','right');
  Mux1 : Mux  Inputs=2
  Mux2 : Mux  Inputs=2
  Mux3 : Mux  Inputs=2
  Saturation1 : Saturate  UpperLimit=5000  LowerLimit=0  RndMeth=Zero
      settings: AttributesFormatString=<limits=%<UpperLimit>/%<LowerLimit>>
  Saturation2 : Saturate  UpperLimit=5000  LowerLimit=0  RndMeth=Zero
      settings: AttributesFormatString=<limits=%<UpperLimit>/%<LowerLimit>>
  Sum1 : Sum  OutDataTypeStr=Inherit: Inherit via back propagation  RndMeth=Zero  InputSameDT=on
  Sum3 : Sum  Inputs=+-  OutDataTypeStr=Inherit: Inherit via back propagation  RndMeth=Zero  InputSameDT=on
  Sum4 : Sum  OutDataTypeStr=Inherit: Inherit via back propagation  RndMeth=Zero  InputSameDT=on
  Vxt_cyl_fill_mdl_pump_mass : Outport
  Vxt_cyl_fill_mdl_ovlp_mass : Outport  Port=2
  Vxt_cyl_igr_mass : Outport  Port=3
  Vxx_cyl_fill_mdl_intk_mfld_prs_cor : Outport  Port=4
  Vxx_cyl_fill_mdl_intk_mfld_prs_diff_cor : Outport  Port=5
  Vxx_cyl_fill_mdl_ex_mfld_prs_rat_cor : Outport  Port=6
  wires:
  Vxx_vvt_ex_angl_cls/1 -> B15_In_cylinder_evc_mass/3(Vxx_vvt_ex_angl_cls)
  Vxx_vvt_ex_angl/1 -> B14_In_cylinder_overlap_mass/4(Vxx_vvt_ex_angl)
  Vxx_intk_vlv_temp/1 -> B13_In_cylinder_ivc_mass/1(Vxx_intk_vlv_temp), B11_Normalization_factor/1(Vxx_intk_vlv_temp)
  Vxx_ex_mfld_temp/1 -> B11_Normalization_factor/2(Vxx_ex_mfld_temp)
  B14_In_cylinder_overlap_mass/1(Vxt_cyl_fill_mdl_ovlp_mass_bas_gas) -> Sum4/1
  Vxx_vvt_intk_angl_cls/1 -> B13_In_cylinder_ivc_mass/4(Vxx_vvt_intk_angl_cls)
  Sum3/1 -> Saturation2/1
  Vxx_vvt_intk_angl_cls_l_lift/1 -> B13_In_cylinder_ivc_mass/5(Vxx_vvt_intk_angl_cls_l_lift)
  Sum1/1 -> Saturation1/1
  B11_Normalization_factor/1(Vxx_cyl_fill_mdl_mass_cor_fac) -> B15_In_cylinder_evc_mass/4(Vxx_cyl_fill_mdl_mass_cor_fac), B14_In_cylinder_overlap_mass/5(Vxx_cyl_fill_mdl_mass_cor_fac)
  Vxx_avg_eng_spd/1 -> B15_In_cylinder_evc_mass/1(Vxx_avg_eng_spd), B14_In_cylinder_overlap_mass/1(Vxx_avg_eng_spd), B13_In_cylinder_ivc_mass/2(Vxx_avg_eng_spd), B12_Exhaust_pressure_correction/6(Vxx_avg_eng_spd)
  B15_In_cylinder_evc_mass/2(Vxt_cyl_fill_mdl_ex_vlv_cls_mass_gas) -> Sum1/2
  Vxx_vvt_intk_angl/1 -> B14_In_cylinder_overlap_mass/3(Vxx_vvt_intk_angl)
  Saturation1/1 -> AEMS_INTERP2/3  "Vxt_cyl_igr_mass_gas"
  B13_In_cylinder_ivc_mass/1(Vxt_cyl_fill_mdl_tot_mass_bas_gas) -> Sum3/1
  B15_In_cylinder_evc_mass/1(Vxt_cyl_fill_mdl_ex_vlv_cls_mass_bas_gas) -> Sum4/2
  Sum4/1 -> Sum3/2
  Vxx_intk_mfld_prs/1 -> B13_In_cylinder_ivc_mass/3(Vxx_intk_mfld_prs), B14_In_cylinder_overlap_mass/2(Vxx_intk_mfld_prs), B15_In_cylinder_evc_mass/2(Vxx_intk_mfld_prs), B12_Exhaust_pressure_correction/5(Vxx_intk_mfld_prs)
  B12_Exhaust_pressure_correction/1(Vxx_cyl_fill_mdl_intk_mfld_prs_diff_cor) -> Vxx_cyl_fill_mdl_intk_mfld_prs_diff_cor/1, B14_In_cylinder_overlap_mass/6(Vxx_cyl_fill_mdl_intk_mfld_prs_diff_cor)
  B12_Exhaust_pressure_correction/2(Vxx_cyl_fill_mdl_ex_mfld_prs_rat_cor) -> B15_In_cylinder_evc_mass/5(Vxx_cyl_fill_mdl_ex_mfld_prs_rat_cor), Vxx_cyl_fill_mdl_ex_mfld_prs_rat_cor/1
  Vxx_atm_prs/1 -> B12_Exhaust_pressure_correction/1(Vxx_atm_prs)
  Vxx_ex_mfld_prs/1 -> B12_Exhaust_pressure_correction/3(Vxx_ex_mfld_prs)
  Vxx_pft_rel_diff_prs/1 -> B12_Exhaust_pressure_correction/2(Vxx_pft_rel_diff_prs)
  Vxx_mdl_ref_ex_mfld_prs/1 -> B12_Exhaust_pressure_correction/4(Vxx_mdl_ref_ex_mfld_prs)
  Saturation2/1 -> AEMS_INTERP1/3  "Vxt_cyl_fill_mdl_pump_mass_bas_gas"
  Mux2/1 -> AEMS_INTERP1/1
  B14_In_cylinder_overlap_mass/2(Vxt_cyl_fill_mdl_ovlp_mass_gas) -> Sum1/1, AEMS_INTERP/3
  Vxx_cyl_fill_mdl_pump_mass_bas_bifuel/1 -> Mux2/2, Mux2/1
  AEMS_INTERP1/1 -> B16_Thermal_corection/1(Vxt_cyl_fill_mdl_pump_mass_bas)  "Vxt_cyl_fill_mdl_pump_mass_bas"
  AEMS_INTERP/1 -> Vxt_cyl_fill_mdl_ovlp_mass/1  "Vxt_cyl_fill_mdl_ovlp_mass"
  AEMS_INTERP2/1 -> Vxt_cyl_igr_mass/1  "Vxt_cyl_igr_mass"
  Vxx_cyl_fill_efy_temp_cor/1 -> B16_Thermal_corection/3(Vxx_cyl_fill_efy_temp_cor)
  B16_Thermal_corection/1(Vxt_cyl_fill_mdl_pump_mass) -> Vxt_cyl_fill_mdl_pump_mass/1
  Vxx_cyl_fill_efy_dyn_cor/1 -> B16_Thermal_corection/2(Vxx_cyl_fill_efy_dyn_cor)
  Vxx_tq_fuel_typ_rat/1 -> AEMS_INTERP/2, AEMS_INTERP2/2, AEMS_INTERP1/2
  Vxx_cyl_fill_mdl_ovlp_mass_bifuel/1 -> Mux1/2, Mux1/1
  Mux1/1 -> AEMS_INTERP/1
  Vxx_cyl_igr_mass_bifuel/1 -> Mux3/2, Mux3/1
  Mux3/1 -> AEMS_INTERP2/1
  B12_Exhaust_pressure_correction/3(Vxx_cyl_fill_mdl_intk_mfld_prs_cor) -> Vxx_cyl_fill_mdl_intk_mfld_prs_cor/1

== system Test_Model_HR12_2016/ASXX_MWIN_FLW_G/ASXX_MWIN_FLW_G/ASXX_MWIN_FLW_filupxxxxg/ASXX_MWIN_FLW_filupxxxxg_10ms/B_Optional_air_filling_estimation/B2_Optional_cylinder_filling_efficiency ==
  Vxx_intk_mfld_prs : Inport  Interpolate=off
  Vxx_intk_vlv_temp : Inport  Port=2  Interpolate=off
  Vxt_cyl_fill_mdl_pump_mass : Inport  Port=3  Interpolate=off
  AEMS_PROTECTED_DIVISION1 : AEMS_Standard_Library/MATH/AEMS_PROTECTED_DIVISION  Tag=[LIB]  out_mode=Default_Output -> Output  tolerance=1
      settings: AttributesFormatString=%<MaskType>\nOutput when |Denominator| < Tolerance = %<out_mode>\nDenominator Tolerance = %<tolerance>
  Calibration2 : Constant  Value=1e+6  OutDataTypeStr=single
  Constant : Constant  Value=0  OutDataTypeStr=single
  Cxx_cyl_nr3 : Constant  Value=Cnx_cyl_nr_conf
  Cxx_cyl_vol : Constant  Value=Cxx_cyl_vol
  Nxx_k_degc : Constant  Value=Nxx_k_degc
  Nxx_k_degc1 : Constant  Value=Nxx_kilo_bas
  Nxx_wht_pgc1 : Constant  Value=Nxx_wht_pgc_j_kg
  Product{6,8,11..12} (4 alike) : Product  Inputs=**  OutDataTypeStr=Inherit: Inherit via back propagation  RndMeth=Zero
  Product14 : Product  Inputs=/*  OutDataTypeStr=Inherit: Inherit via back propagation  RndMeth=Zero
  Product7 : Product  Inputs=*/  OutDataTypeStr=Inherit: Inherit via back propagation  RndMeth=Zero
  Saturation1 : Saturate  UpperLimit=2  LowerLimit=0  RndMeth=Zero
      settings: AttributesFormatString=<limits=%<UpperLimit>/%<LowerLimit>>
  Saturation2 : Saturate  UpperLimit=12  LowerLimit=3  RndMeth=Zero
      settings: AttributesFormatString=<limits=%<UpperLimit>/%<LowerLimit>>
  Saturation3 : Saturate  UpperLimit=135794.05  LowerLimit=66914.05  RndMeth=Zero
      settings: AttributesFormatString=<limits=%<UpperLimit>/%<LowerLimit>>
  Sum2 : Sum  OutDataTypeStr=Inherit: Inherit via back propagation  RndMeth=Zero  InputSameDT=on
  Vxt_cyl_fill_efy_opt : Outport
  wires:
  Cxx_cyl_vol/1 -> Product7/1
  Product8/1 -> Product11/1
  Sum2/1 -> Product6/1
  Nxx_k_degc/1 -> Sum2/2
  Vxx_intk_vlv_temp/1 -> Sum2/1
  Product6/1 -> Saturation3/1
  Product11/1 -> Product14/2
  Nxx_k_degc1/1 -> Product8/2
  Product7/1 -> Product11/2
  Nxx_wht_pgc1/1 -> Product6/2
  Cxx_cyl_nr3/1 -> Saturation2/1
  Saturation1/1 -> Vxt_cyl_fill_efy_opt/1  "Vxt_cyl_fill_efy_opt"
  Vxx_intk_mfld_prs/1 -> Product8/1
  AEMS_PROTECTED_DIVISION1/1 -> Saturation1/1
  Saturation2/1 -> Product7/2
  Saturation3/1 -> Product14/1
  Calibration2/1 -> Product12/2
  Product12/1 -> AEMS_PROTECTED_DIVISION1/2
  Vxt_cyl_fill_mdl_pump_mass/1 -> AEMS_PROTECTED_DIVISION1/1
  Product14/1 -> Product12/1
  Constant/1 -> AEMS_PROTECTED_DIVISION1/3

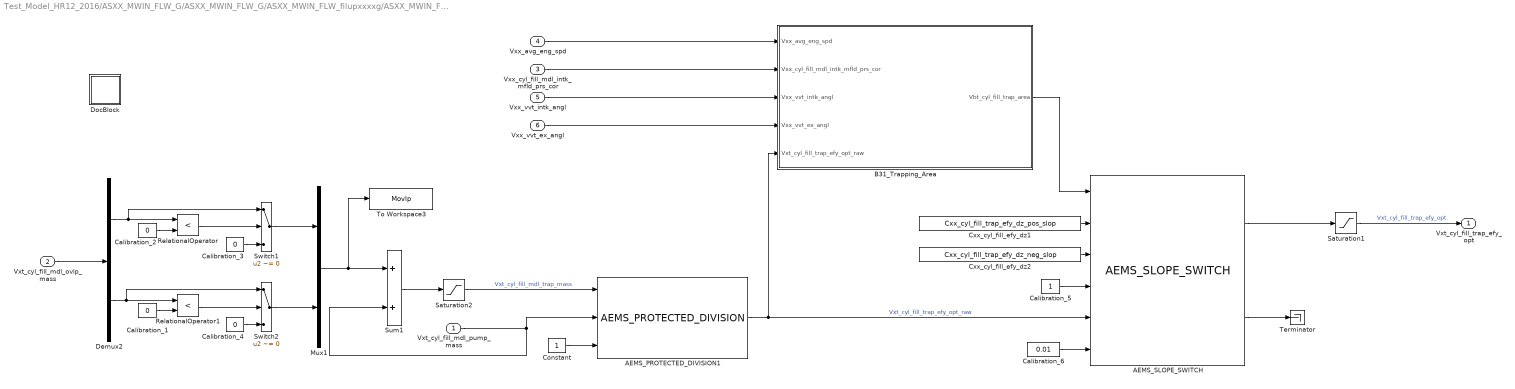
== system Test_Model_HR12_2016/ASXX_MWIN_FLW_G/ASXX_MWIN_FLW_G/ASXX_MWIN_FLW_filupxxxxg/ASXX_MWIN_FLW_filupxxxxg_10ms/B_Optional_air_filling_estimation/B3_Optional_cylinder_trapping_efficiency ==
  Vxt_cyl_fill_mdl_pump_mass : Inport  Interpolate=off
  Vxt_cyl_fill_mdl_ovlp_mass : Inport  Port=2  Interpolate=off
  Vxx_cyl_fill_mdl_intk_mfld_prs_cor : Inport  Port=3  Interpolate=off
  Vxx_avg_eng_spd : Inport  Port=4  Interpolate=off
  Vxx_vvt_intk_angl : Inport  Port=5  Interpolate=off
  Vxx_vvt_ex_angl : Inport  Port=6  Interpolate=off
  AEMS_PROTECTED_DIVISION1 : AEMS_Standard_Library/MATH/AEMS_PROTECTED_DIVISION  Tag=[LIB]  out_mode=Default_Output -> Output  tolerance=10
      settings: AttributesFormatString=%<MaskType>\nOutput when |Denominator| < Tolerance = %<out_mode>\nDenominator Tolerance = %<tolerance>
  AEMS_SLOPE_SWITCH : AEMS_Standard_Library/DISCONTINUITIES/AEMS_SLOPE_SWITCH  Tag=[LIB]
      settings: AttributesFormatString=%<MaskType>
  B31_Trapping_Area : Subsystem
  Calibration_1 : Constant  Value=0
  Calibration_2 : Constant  Value=0
  Calibration_3 : Constant  Value=0  LockScale=on
  Calibration_4 : Constant  Value=0  OutDataTypeStr=Inherit: Inherit via back propagation
  Calibration_5 : Constant
  Calibration_6 : Constant  Value=0.01
  Constant : Constant  OutDataTypeStr=single
  Cxx_cyl_fill_efy_dz1 : Constant  Value=Cxx_cyl_fill_trap_efy_dz_pos_slop
  Cxx_cyl_fill_efy_dz2 : Constant  Value=Cxx_cyl_fill_trap_efy_dz_neg_slop
  Demux2 : Demux  Outputs=2
  DocBlock : Subsystem  InitFcn=docblock('save_document',gcb);  mask(DocBlock){ECoderFlag=, DocumentType=RTF}
      mask prompts: ECoderFlag "Simulink:masks:DocBlockEmbeddedCoderFlagLabel_MP"; DocumentType "Simulink:masks:DocBlockDocTypeLabel_MP"
      mask help: Simulink:masks:DocBlock_MD
      settings: DeleteFcn=docblock('close_document',gcb);  PreSaveFcn=docblock('save_document',gcb);  OpenFcn=docblock('edit_document',gcb);
      mask TypeOptions DocumentType: Simulink:masks:Text | Simulink:masks:RTF | Simulink:masks:HTML
      mask Display:
      | plot([.8 0 0 1 1 .8 .8 1],[1 1 0 0 .8 1 .8 .8]);
      | text(.5,.6,'DOC','horizontalalignment','center');
      | text(.95,.05,get_param(gcb,'DocumentType'),'verticalalignment','bottom','horizontalalignment','right');
  Mux1 : Mux  Inputs=2
  RelationalOperator : RelationalOperator  Operator=<  OutDataTypeStr=boolean  RndMeth=Nearest  InputSameDT=on
  RelationalOperator1 : RelationalOperator  Operator=<  OutDataTypeStr=boolean  RndMeth=Nearest  InputSameDT=on
  Saturation1 : Saturate  UpperLimit=2  LowerLimit=0  RndMeth=Zero
      settings: AttributesFormatString=<limits=%<UpperLimit>/%<LowerLimit>>
  Saturation2 : Saturate  UpperLimit=5000  LowerLimit=0  RndMeth=Zero
      settings: AttributesFormatString=<limits=%<UpperLimit>/%<LowerLimit>>
  Sum1 : Sum  OutDataTypeStr=Inherit: Inherit via back propagation  RndMeth=Zero  InputSameDT=on
  Switch1 : Switch  Criteria=u2 ~= 0  RndMeth=Zero  SaturateOnIntegerOverflow=on  InputSameDT=on
      settings: AttributesFormatString=Criteria=%<Criteria>
  Switch2 : Switch  Criteria=u2 ~= 0  RndMeth=Zero  SaturateOnIntegerOverflow=on  InputSameDT=on
      settings: AttributesFormatString=Criteria=%<Criteria>
  Terminator : Terminator
  To Workspace3 : ToWorkspace  VariableName=Movlp  SampleTime=1
  Vxt_cyl_fill_trap_efy_opt : Outport
  wires:
  Vxt_cyl_fill_mdl_ovlp_mass/1 -> Demux2/1
  Calibration_2/1 -> RelationalOperator/2
  Calibration_1/1 -> RelationalOperator1/2
  RelationalOperator/1 -> Switch1/2
  RelationalOperator1/1 -> Switch2/2
  Demux2/1 -> Switch1/1, RelationalOperator/1
  Demux2/2 -> Switch2/1, RelationalOperator1/1
  Calibration_3/1 -> Switch1/3
  Calibration_4/1 -> Switch2/3
  Switch1/1 -> Mux1/1
  Switch2/1 -> Mux1/2
  AEMS_SLOPE_SWITCH/1 -> Saturation1/1
  Saturation1/1 -> Vxt_cyl_fill_trap_efy_opt/1  "Vxt_cyl_fill_trap_efy_opt"
  Mux1/1 -> To Workspace3/1, Sum1/1
  Sum1/1 -> Saturation2/1
  Vxt_cyl_fill_mdl_pump_mass/1 -> Sum1/2, AEMS_PROTECTED_DIVISION1/2
  Saturation2/1 -> AEMS_PROTECTED_DIVISION1/1  "Vxt_cyl_fill_mdl_trap_mass"
  Calibration_6/1 -> AEMS_SLOPE_SWITCH/6
  Calibration_5/1 -> AEMS_SLOPE_SWITCH/4
  Cxx_cyl_fill_efy_dz1/1 -> AEMS_SLOPE_SWITCH/2
  Cxx_cyl_fill_efy_dz2/1 -> AEMS_SLOPE_SWITCH/3
  AEMS_SLOPE_SWITCH/2 -> Terminator/1
  AEMS_PROTECTED_DIVISION1/1 -> AEMS_SLOPE_SWITCH/5, B31_Trapping_Area/5(Vxt_cyl_fill_trap_efy_opt_raw)  "Vxt_cyl_fill_trap_efy_opt_raw"
  Constant/1 -> AEMS_PROTECTED_DIVISION1/3
  Vxx_avg_eng_spd/1 -> B31_Trapping_Area/1(Vxx_avg_eng_spd)
  Vxx_cyl_fill_mdl_intk_mfld_prs_cor/1 -> B31_Trapping_Area/2(Vxx_cyl_fill_mdl_intk_mfld_prs_cor)
  Vxx_vvt_intk_angl/1 -> B31_Trapping_Area/3(Vxx_vvt_intk_angl)
  Vxx_vvt_ex_angl/1 -> B31_Trapping_Area/4(Vxx_vvt_ex_angl)
  B31_Trapping_Area/1(Vbt_cyl_fill_trap_area) -> AEMS_SLOPE_SWITCH/1

== system Test_Model_HR12_2016/ASXX_MWIN_FLW_G/ASXX_MWIN_FLW_G/ASXX_MWIN_FLW_filupxxxxg/ASXX_MWIN_FLW_filupxxxxg_10ms/C_consolidation/C1_filter_for_throttle_command ==
  Vxt_cyl_fill_efy : Inport  Interpolate=off
  AEMS_DEADZONE1 : AEMS_Standard_Library/DISCONTINUITIES/AEMS_DEADZONE  Tag=[LIB]  mf=on
      settings: AttributesFormatString=%<MaskType>\nCurve inflexion dead-zone = %<mf>
  AEMS_SlewRate2_v02_00 : AEMS_Standard_Library/DISCONTINUITIES/AEMS_SLEW_RATE  Tag=[LIB]
      settings: AttributesFormatString=%<MaskType>
  Constant : Constant  Value=0.01  OutDataTypeStr=single
  Constant1 : Constant  Value=-1  OutDataTypeStr=single
  Constant2 : Constant  Value=-1  OutDataTypeStr=single
  Cxx_cyl_fill_efy_drv_max : Constant  Value=Cxx_cyl_fill_efy_drv_max
  Cxx_cyl_fill_efy_dz : Constant  Value=Cxx_cyl_fill_efy_dz
  DocBlock : Subsystem  mask(DocBlock){ECoderFlag=, DocumentType=Text}
      mask prompts: ECoderFlag "Simulink:blocks:docblockEmbeddedCoderFlagLabel"; DocumentType "Simulink:blocks:docblockDocTypeLabel"
      mask help: Use this block to save long descriptive text with the model. Double-clicking the block will open an editor.
      mask TypeOptions DocumentType: Text | RTF | HTML
      mask Display:
      | plot([.8 0 0 1 1 .8 .8 1],[1 1 0 0 .8 1 .8 .8]);
      | text(.5,.6,'DOC','horizontalalignment','center');
      | text(.95,.05,get_param(gcb,'DocumentType'),'verticalalignment','bottom','horizontalalignment','right');
  Product : Product  OutDataTypeStr=Inherit: Inherit via back propagation  RndMeth=Zero
  Product1 : Product  OutDataTypeStr=Inherit: Inherit via back propagation  RndMeth=Zero
  Saturation2 : Saturate  UpperLimit=2  LowerLimit=0  RndMeth=Zero
      settings: AttributesFormatString=<limits=%<UpperLimit>/%<LowerLimit>>
  Vxt_cyl_fill_efy_fil : Outport
  wires:
  Constant/1 -> AEMS_SlewRate2_v02_00/4
  Vxt_cyl_fill_efy/1 -> AEMS_SlewRate2_v02_00/2
  AEMS_SlewRate2_v02_00/1 -> AEMS_DEADZONE1/1
  Product/1 -> AEMS_SlewRate2_v02_00/3
  Constant1/1 -> Product/2
  Cxx_cyl_fill_efy_dz/1 -> AEMS_DEADZONE1/3, Product1/1
  Product1/1 -> AEMS_DEADZONE1/2
  AEMS_DEADZONE1/1 -> Saturation2/1
  Constant2/1 -> Product1/2
  Cxx_cyl_fill_efy_drv_max/1 -> Product/1, AEMS_SlewRate2_v02_00/1
  Saturation2/1 -> Vxt_cyl_fill_efy_fil/1  "Vxt_cyl_fill_efy_fil"

== system Test_Model_HR12_2016/ASXX_MWIN_FLW_G/ASXX_MWIN_FLW_G/ASXX_MWIN_FLW_filupxxxxg/ASXX_MWIN_FLW_filupxxxxg_10ms/DocBlock/EmptySubsystem ==

== system Test_Model_HR12_2016/ASXX_MWIN_FLW_G/ASXX_MWIN_FLW_G/ASXX_MWIN_FLW_pumpflwxxg/ASXX_MWIN_FLW_pumpflwxxg_10ms/DocBlock/EmptySubsystem ==

== system Test_Model_HR12_2016/ASXX_MWIN_FLW_G/ASXX_MWIN_FLW_G/ASXX_MWIN_FLW_pzeroxxxxg/ASXX_MWIN_FLW_pzeroxxxxg_10ms/DocBlock/EmptySubsystem ==

== system Test_Model_HR12_2016/ASXX_MWIN_FLW_G/ASXX_MWIN_FLW_G/ASXX_MWIN_FLW_trapexxxxg/ASXX_MWIN_FLW_trapexxxxg_10ms/DocBlock/EmptySubsystem ==

== system Test_Model_HR12_2016/ASXX_MWIN_FLW_G/ASXX_MWIN_FLW_G/ASXX_MWIN_FLW_trapexxxxg/ASXX_MWIN_FLW_trapexxxxg_10ms/Trapexxxxg/B1_crossing_position_correction ==
  Vxx_avg_eng_spd : Inport  Interpolate=off
  Vxx_cyl_fill_efy_intk_mfld_prs_atm_prs_cor : Inport  Port=2  Interpolate=off
  Vxx_vvt_ex_angl : Inport  Port=3  Interpolate=off
  Vxx_vvt_intk_angl : Inport  Port=4  Interpolate=off
  AEMS_Carto_2D_v01_02 : AEMS_Standard_Library/LOOKUP_TABLES/AEMS_LUT_2D  Tag=[LIB]  map_x=Cxb_cyl_fill_eng_spd  map_y=Cxb_cyl_fill_intk_mfld_prs  carto=Cxm_cyl_fill_trap_efy_vvt_ovlp_psn_cor_fac_1
      settings: AttributesFormatString=%<MaskType>\nBkPX=%<map_x>\nBkPY=%<map_y>\nMAP=%<carto>
  AEMS_Carto_2D_v01_1 : AEMS_Standard_Library/LOOKUP_TABLES/AEMS_LUT_2D  Tag=[LIB]  map_x=Cxb_cyl_fill_eng_spd  map_y=Cxb_cyl_fill_intk_mfld_prs  carto=Cxm_cyl_fill_trap_efy_vvt_ovlp_psn_cor_fac_2
      settings: AttributesFormatString=%<MaskType>\nBkPX=%<map_x>\nBkPY=%<map_y>\nMAP=%<carto>
  Constant2 : Constant  Value=2  OutDataTypeStr=single
  Constant3 : Constant  Value=0  OutDataTypeStr=single
  Cxx_cyl_fill_trap_vvt_ovlp_angl : Constant  Value=Cxx_cyl_fill_trap_vvt_ovlp_angl
  Divide : Product  Inputs=*/  OutDataTypeStr=Inherit: Inherit via back propagation  RndMeth=Zero
  DocBlock : Subsystem  mask(DocBlock){ECoderFlag=, DocumentType=RTF}
      mask prompts: ECoderFlag "Simulink:blocks:docblockEmbeddedCoderFlagLabel"; DocumentType "Simulink:blocks:docblockDocTypeLabel"
      mask help: Use this block to save long descriptive text with the model. Double-clicking the block will open an editor.
      mask TypeOptions DocumentType: Text | RTF | HTML
      mask Display:
      | plot([.8 0 0 1 1 .8 .8 1],[1 1 0 0 .8 1 .8 .8]);
      | text(.5,.6,'DOC','horizontalalignment','center');
      | text(.95,.05,get_param(gcb,'DocumentType'),'verticalalignment','bottom','horizontalalignment','right');
  Product1 : Product  OutDataTypeStr=Inherit: Inherit via back propagation  RndMeth=Zero
  Product3 : Product  OutDataTypeStr=Inherit: Inherit via back propagation  RndMeth=Zero
  Product4 : Product  OutDataTypeStr=Inherit: Inherit via back propagation  RndMeth=Zero
  RelationalOperator : RelationalOperator  OutDataTypeStr=boolean  RndMeth=Nearest  InputSameDT=on
  Saturation : Saturate  UpperLimit=1  LowerLimit=-1  RndMeth=Zero
      settings: AttributesFormatString=<limits=%<UpperLimit>/%<LowerLimit>>
  Sum1 : Sum  Inputs=-+  OutDataTypeStr=Inherit: Inherit via back propagation  RndMeth=Zero  InputSameDT=on
  Sum2 : Sum  OutDataTypeStr=Inherit: Inherit via back propagation  RndMeth=Zero  InputSameDT=on
  Sum4 : Sum  Inputs=+-  OutDataTypeStr=Inherit: Inherit via back propagation  RndMeth=Zero  InputSameDT=on
  Switch : Switch  Criteria=u2 ~= 0  RndMeth=Zero  SaturateOnIntegerOverflow=on  InputSameDT=on
      settings: AttributesFormatString=Criteria=%<Criteria>
  Vxx_cyl_fill_trap_efy_vvt_ovlp_psn_cor : Outport
  wires:
  AEMS_Carto_2D_v01_1/1 -> Product1/2  "Vxx_cyl_fill_trap_efy_vvt_ovlp_psn_cor_fac_2"
  Vxx_cyl_fill_efy_intk_mfld_prs_atm_prs_cor/1 -> AEMS_Carto_2D_v01_1/2, AEMS_Carto_2D_v01_02/2
  Vxx_avg_eng_spd/1 -> AEMS_Carto_2D_v01_02/1, AEMS_Carto_2D_v01_1/1
  AEMS_Carto_2D_v01_02/1 -> Product4/1  "Vxx_cyl_fill_trap_efy_vvt_ovlp_psn_cor_fac_1"
  Divide/1 -> Switch/1
  Constant2/1 -> Divide/2
  Sum4/1 -> Divide/1
  Switch/1 -> Product1/1, Product3/1, Product3/2
  Sum1/1 -> Saturation/1
  Product4/1 -> Sum1/1
  Product1/1 -> Sum1/2
  Vxx_vvt_ex_angl/1 -> Sum2/1, Sum4/2
  Vxx_vvt_intk_angl/1 -> Sum4/1, Sum2/2
  Sum2/1 -> RelationalOperator/1
  Cxx_cyl_fill_trap_vvt_ovlp_angl/1 -> RelationalOperator/2
  RelationalOperator/1 -> Switch/2
  Constant3/1 -> Switch/3
  Product3/1 -> Product4/2
  Saturation/1 -> Vxx_cyl_fill_trap_efy_vvt_ovlp_psn_cor/1  "Vxx_cyl_fill_trap_efy_vvt_ovlp_psn_cor"
